simulink model "code_withlinear_addition_at_receiver"  (R2016b)
settings: Solver=VariableStepAuto  StartTime=0.0  StopTime=10.0  RelTol=1e-3
undefined symbols (not defined in the file or in its folder): doppler, physconst
libraries: phasedenvlib x12, phasedtxrxlib x7, commchan3 x4, dspinverses x4
settings Model: Creator=CHAITRA  LastModifiedBy=CHAITRA

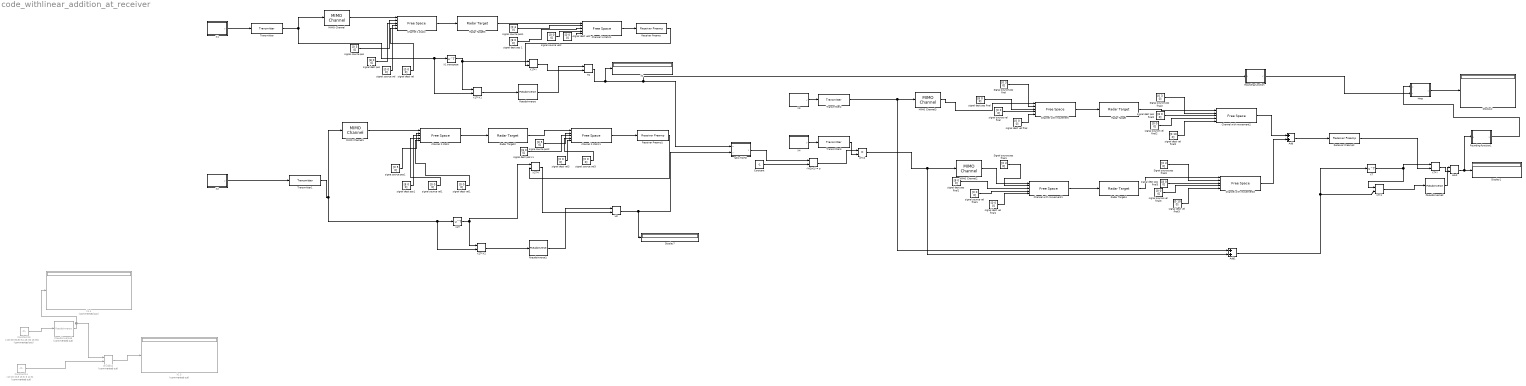
== system code_withlinear_addition_at_receiver ==
  -(H2/H1) = p : Product  Multiplication=Matrix(*)
  Add : Sum
  Add1 : Sum
  Channel 1 static : phasedenvlib/Free Space  PropagationSpeed=physconst( 'LightSpeed' )  OperatingFrequency=3e8  TwoWayPropagation=off  SampleRateFromInputCheckbox=off  SampleRate=100  MaximumDistanceSource=Property  MaximumDistance=10  MaximumNumInputSamplesSource=Auto  MaximumNumInputSamples=1000  SimulateUsing=Interpreted execution
  Channel 1 static1 : phasedenvlib/Free Space  PropagationSpeed=physconst( 'LightSpeed' )  OperatingFrequency=3e8  TwoWayPropagation=off  SampleRateFromInputCheckbox=off  SampleRate=100  MaximumDistanceSource=Property  MaximumDistance=10  MaximumNumInputSamplesSource=Auto  MaximumNumInputSamples=1000  SimulateUsing=Interpreted execution
  Channel with movement{,1..3} (4 alike) : phasedenvlib/Free Space  PropagationSpeed=physconst( 'LightSpeed' )  OperatingFrequency=3e8  TwoWayPropagation=off  SampleRateFromInputCheckbox=off  SampleRate=100  MaximumDistanceSource=Property  MaximumDistance=10  MaximumNumInputSamplesSource=Auto  MaximumNumInputSamples=1000  SimulateUsing=Interpreted execution
  Constant : Constant  Value=-1
  Constant13 : Constant  Commented=on  Value=[100 80 60;80 64 48; 60 48 36]
  Constant14 : Constant  Commented=on  Value=[10 20 10;8 16 8; 6 12 6]
  Display1 : Display
  Display2 : Display
  Display7 : Display
  Divide11 : Product  Commented=on  Multiplication=Matrix(*)
  H1 : Product  Multiplication=Matrix(*)
  H2 : Product  Multiplication=Matrix(*)
  Hout : Product  Multiplication=Matrix(*)
  "Hres " : MATLAB Function  TreatAsAtomicUnit=on
  MIMO Channel{,1..3} (4 alike) : commchan3/MIMO Channel  SampleRate=100  PathDelays=0  AveragePathGains=0  NormalizePathGains=on  FadingDistribution=Rayleigh  KFactor=3  DirectPathDopplerShift=0  DirectPathInitialPhase=0  MaximumDopplerShift=0.001  DopplerSpectrum=doppler( 'Jakes' )  SpatialCorrelation=off  NumTransmitAntennas=1  NumReceiveAntennas=1  TransmitCorrelationMatrix=[1 0; 0 1]  ReceiveCorrelationMatrix=[1 0; 0 1]  AntennaSelection=Off  NormalizeChannelOutputs=on  SimulateUsing=Interpreted execution  FadingTechnique=Filtered Gaussian noise  NumSinusoids=48  InitialTimeSource=Property  InitialTime=0  RandomStream=mt19937ar with seed  Seed=73  PathGainsOutputPort=off  Visualization=Off  AntennaPairsToDisplay=[ 1, 1 ]  PathsForDopplerDisplay=1  SamplesToDisplay=25%
  Pseudoinverse : dspinverses/Pseudoinverse  wanterr=off  SimulateUsing=Interpreted execution
  Pseudoinverse1 : dspinverses/Pseudoinverse  wanterr=off  SimulateUsing=Interpreted execution
  Pseudoinverse2 : dspinverses/Pseudoinverse  wanterr=off  SimulateUsing=Interpreted execution
  Pseudoinverse3 : dspinverses/Pseudoinverse  Commented=on  wanterr=off  SimulateUsing=Interpreted execution
  Radar Target{,2..4} (4 alike) : phasedenvlib/Radar Target  EnablePolarization=off  Mode=Monostatic  MeanRCSSource=Property  ScatteringMatrixSource=Property  MeanRCS=1  ScatteringMatrix=eye( 2 )  Model=Nonfluctuating  PropagationSpeed=physconst( 'LightSpeed' )  OperatingFrequency=3e8  SeedSource=Property  Seed=randi(65535,1)  SimulateUsing=Interpreted execution
  Receiver Preamp : phasedtxrxlib/Receiver Preamp  Gain=20  LossFactor=0  NoiseMethod=Noise power  NoiseFigure=0  ReferenceTemperature=290  SampleRateFromInputCheckbox=on  SampleRate=1e6  NoisePower=0  EnableInputPort=off  PhaseNoiseInputPort=off  SeedSource=Property  Seed=randi(65535,1)  SimulateUsing=Interpreted execution
  Receiver Preamp1 : phasedtxrxlib/Receiver Preamp  Gain=20  LossFactor=0  NoiseMethod=Noise power  NoiseFigure=0  ReferenceTemperature=290  SampleRateFromInputCheckbox=on  SampleRate=1e6  NoisePower=0  EnableInputPort=off  PhaseNoiseInputPort=off  SeedSource=Property  Seed=randi(65535,1)  SimulateUsing=Interpreted execution
  Receiver Preamp2 : phasedtxrxlib/Receiver Preamp  Gain=20  LossFactor=0  NoiseMethod=Noise power  NoiseFigure=0  ReferenceTemperature=290  SampleRateFromInputCheckbox=on  SampleRate=1e6  NoisePower=0  EnableInputPort=off  PhaseNoiseInputPort=off  SeedSource=Property  Seed=randi(65535,1)  SimulateUsing=Interpreted execution
  Rounding function : MATLAB Function  TreatAsAtomicUnit=on
  Rounding function1 : MATLAB Function  TreatAsAtomicUnit=on
  Signal source pos final{,1..3} (4 alike) : Constant  Value=[0 3 0]
  Transmitter{,1..3} (4 alike) : phasedtxrxlib/Transmitter  PeakPower=5000  Gain=20  LossFactor=0  InUseOutputPort=off  CoherentOnTransmit=on  PhaseNoiseOutputPort=off  SeedSource=Property  Seed=randi(65535,1)  SimulateUsing=Interpreted execution
  X1 : MATLAB Function  TreatAsAtomicUnit=on
  X1 transpose : Math  Operator=transpose  SaturateOnIntegerOverflow=on
  X1T*X1 : Product  Multiplication=Matrix(*)
  X1T*Y : Product  Multiplication=Matrix(*)
  X2 : MATLAB Function  TreatAsAtomicUnit=on
  X2T : Math  Operator=transpose  SaturateOnIntegerOverflow=on
  X2T*X2 : Product  Multiplication=Matrix(*)
  X2T*Y : Product  Multiplication=Matrix(*)
  X3 : MATLAB Function  TreatAsAtomicUnit=on
  X4 : MATLAB Function  TreatAsAtomicUnit=on
  XT : Math  Operator=transpose  SaturateOnIntegerOverflow=on
  XT*X : Product  Multiplication=Matrix(*)
  XT*Y : Product  Multiplication=Matrix(*)
  channel 2 static : phasedenvlib/Free Space  PropagationSpeed=physconst( 'LightSpeed' )  OperatingFrequency=3e8  TwoWayPropagation=off  SampleRateFromInputCheckbox=off  SampleRate=100  MaximumDistanceSource=Property  MaximumDistance=10  MaximumNumInputSamplesSource=Auto  MaximumNumInputSamples=1000  SimulateUsing=Interpreted execution
  channel 2 static1 : phasedenvlib/Free Space  PropagationSpeed=physconst( 'LightSpeed' )  OperatingFrequency=3e8  TwoWayPropagation=off  SampleRateFromInputCheckbox=off  SampleRate=100  MaximumDistanceSource=Property  MaximumDistance=10  MaximumNumInputSamplesSource=Auto  MaximumNumInputSamples=1000  SimulateUsing=Interpreted execution
  "h1 " : Display
  h1 4 : Display  Commented=on
  h1 5 : Display  Commented=on
  p*X2 : Product
  ratio H1/H2 : MATLAB Function  TreatAsAtomicUnit=on
  signa source pos1 : Constant  Value=[0 5 0]
  signa source pos2 : Constant  Value=[0 5 0]
  "signal dest pos " : Constant  Value=[8 0 0]
  signal dest pos 1 : Constant  Value=[8 0 0]
  signal dest pos final{,1..3} (4 alike) : Constant  Value=[8 0 0]
  "signal dest pos1 " : Constant  Value=[8 0 0]
  signal dest pos1 1 : Constant  Value=[8 0 0]
  signal dest vel{,1..3} (4 alike) : Constant  Value=[0 0 0]
  signal dest vel final : Constant  Value=[0 0 0]
  signal dest vel final1 : Constant  Value=[0 0 0]
  signal dest vel final2 : Constant  Value=[0 10 0]
  signal dest vel final3 : Constant  Value=[0 10 0]
  signal source pos : Constant  Value=[0 3 0]
  signal source pos1 : Constant  Value=[0 3 0]
  signal source vel{,1..3} (4 alike) : Constant  Value=[0 0 0]
  signal source vel final{,1..3} (4 alike) : Constant  Value=[0 0 0]
  wires:
  X1 transpose/1 -> X1T*X1/1, X1T*Y/1
  X1T*X1/1 -> Pseudoinverse/1
  X1T*Y/1 -> H1/2
  ratio H1/H2/1(y) -> -(H2/H1) = p/1
  X1/1(y) -> Transmitter/1
  Receiver Preamp/1 -> X1T*Y/2
  Pseudoinverse/1 -> H1/1
  X2T/1 -> X2T*Y/1, X2T*X2/1
  X2T*X2/1 -> Pseudoinverse1/1
  X2T*Y/1 -> H2/2
  X2/1(y) -> Transmitter1/1
  Receiver Preamp1/1 -> X2T*Y/2
  Pseudoinverse1/1 -> H2/1
  Constant/1 -> -(H2/H1) = p/2
  -(H2/H1) = p/1 -> p*X2/1
  X3/1(y) -> Transmitter2/1
  X4/1(y) -> Transmitter3/1
  Transmitter3/1 -> p*X2/2
  H2/1 -> Display7/1, ratio H1/H2/2(v)
  signal source pos/1 -> Channel 1 static/2
  "signal dest pos "/1 -> Channel 1 static/3
  signal source vel/1 -> Channel 1 static/4
  signal dest vel/1 -> Channel 1 static/5
  signa source pos1/1 -> channel 2 static/2
  "signal dest pos1 "/1 -> channel 2 static/3
  signal source vel1/1 -> channel 2 static/4
  signal dest vel1/1 -> channel 2 static/5
  Signal source pos final/1 -> Channel with movement/2
  signal dest pos final/1 -> Channel with movement/3
  signal source vel final/1 -> Channel with movement/4
  signal dest vel final/1 -> Channel with movement/5
  Constant13/1 -> Pseudoinverse3/1
  Pseudoinverse3/1 -> Divide11/1, h1 4/1
  Constant14/1 -> Divide11/2
  Divide11/1 -> h1 5/1
  Channel 1 static/1 -> Radar Target3/1
  channel 2 static/1 -> Radar Target2/1
  MIMO Channel/1 -> Channel 1 static/1
  MIMO Channel1/1 -> channel 2 static/1
  MIMO Channel3/1 -> Channel with movement/1
  Transmitter/1 -> X1T*X1/2, X1 transpose/1, MIMO Channel/1
  Transmitter1/1 -> MIMO Channel1/1, X2T*X2/2, X2T/1
  signal source pos1/1 -> Channel 1 static1/2
  signal dest pos 1/1 -> Channel 1 static1/3
  signal source vel2/1 -> Channel 1 static1/4
  signal dest vel2/1 -> Channel 1 static1/5
  Radar Target3/1 -> Channel 1 static1/1
  Channel 1 static1/1 -> Receiver Preamp/1
  signa source pos2/1 -> channel 2 static1/2
  signal dest pos1 1/1 -> channel 2 static1/3
  signal source vel3/1 -> channel 2 static1/4
  signal dest vel3/1 -> channel 2 static1/5
  channel 2 static1/1 -> Receiver Preamp1/1
  Radar Target2/1 -> channel 2 static1/1
  Signal source pos final1/1 -> Channel with movement1/2
  signal dest pos final1/1 -> Channel with movement1/3
  signal source vel final1/1 -> Channel with movement1/4
  signal dest vel final1/1 -> Channel with movement1/5
  MIMO Channel2/1 -> Channel with movement1/1
  p*X2/1 -> Add1/2, MIMO Channel2/1
  Transmitter2/1 -> Add1/1, MIMO Channel3/1
  Channel with movement1/1 -> Radar Target4/1
  Channel with movement/1 -> Radar Target/1
  Signal source pos final2/1 -> Channel with movement2/2
  signal dest pos final2/1 -> Channel with movement2/3
  signal source vel final2/1 -> Channel with movement2/4
  signal dest vel final2/1 -> Channel with movement2/5
  Radar Target/1 -> Channel with movement2/1
  Signal source pos final3/1 -> Channel with movement3/2
  signal dest pos final3/1 -> Channel with movement3/3
  signal source vel final3/1 -> Channel with movement3/4
  signal dest vel final3/1 -> Channel with movement3/5
  Radar Target4/1 -> Channel with movement3/1
  Channel with movement2/1 -> Add/1
  Channel with movement3/1 -> Add/2
  Add/1 -> Receiver Preamp2/1
  XT/1 -> XT*X/1, XT*Y/1
  XT*X/1 -> Pseudoinverse2/1
  XT*Y/1 -> Hout/2
  Pseudoinverse2/1 -> Hout/1
  Receiver Preamp2/1 -> XT*Y/2
  Hout/1 -> Rounding function1/1(u), Display1/1
  Add1/1 -> XT*X/2, XT/1
  "Hres "/1(y) -> Display2/1
  H1/1 -> "h1 "/1, Rounding function/1(u), ratio H1/H2/1(u)
  Rounding function/1(y) -> "Hres "/2(v)
  Rounding function1/1(y) -> "Hres "/1(u)

== matlab function code_withlinear_addition_at_receiver/X1 ==
  data: y output
function y = fcn()

f = 800e6;
t = 0:0.01:1;

a = 5*sin(2*pi*f*t);

y = transpose(a);

== matlab function code_withlinear_addition_at_receiver/X2 ==
  data: y output
function y = fcn()

f = 800e6;
t = 0:0.01:1;

a = 5*sin(2*pi*f*t);

y = transpose(a);

== matlab function code_withlinear_addition_at_receiver/X3 ==
  data: y output
function y = fcn()

f = 800e6;
t = 0:0.01:1;

a = 5*sin(2*pi*f*t);

y = transpose(a);

== matlab function code_withlinear_addition_at_receiver/ratio H1//H2 ==
  data: u input; y output; v input
function y = fcn(u,v)

%y = ldivide(w,z)
% you can divide each element by the same eleent of other row by
y= u./v ;

== matlab function code_withlinear_addition_at_receiver/X4 ==
  data: y output
function y = fcn()

f = 800e6;
t = 0:0.01:1;

a = 5*sin(2*pi*f*t);

y = transpose(a);

== matlab function code_withlinear_addition_at_receiver/Hres  ==
  data: u input; y output; v input
function y = fcn(u,v)

%y = ldivide(w,z)
% you can divide each element by the same eleent of other row by
y= u-v ;

== matlab function code_withlinear_addition_at_receiver/Rounding function1 ==
  data: u input; y output
function y = fcn(u)

y = round(u*100000000)/100000000;

== matlab function code_withlinear_addition_at_receiver/Rounding function ==
  data: u input; y output
function y = fcn(u)

y = round(u*100000000)/100000000;
